simulink model "colab_sim"  (R2023b)
settings: Solver=VariableStepAuto  StartTime=0.0  StopTime=20e-3  RelTol=1e-3
values from neighbouring files (symbols this model uses):
  C = single(10e-6)    [colab_datagen.m]
  dt = 1/f_m    (= 1.25e-06)    [colab_datagen.m]
  ESR = 2    [colab_datagen.m]
  L = single(460e-6)    [colab_datagen.m]
  R = randi([18 50])    [colab_datagen.m]
  R_L = 0.75    [colab_datagen.m]
  Vin = 200    [colab_datagen.m]
libraries: spsSeriesRLCBranchLib x3, spsCurrentMeasurementLib x1, spsDCVoltageSourceLib x1, spsDiodeLib x1, spsMosfetLib x1, dspstat3 x1, dspsrcs4 x1, spsVoltageMeasurementLib x1, spspowerguiLib x1
settings Model: Creator=User  LastModifiedBy=User

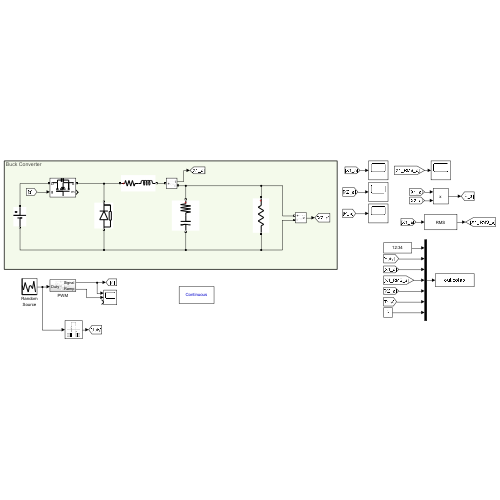
[thumbnail: Simulink's stored preview of the top-level diagram]
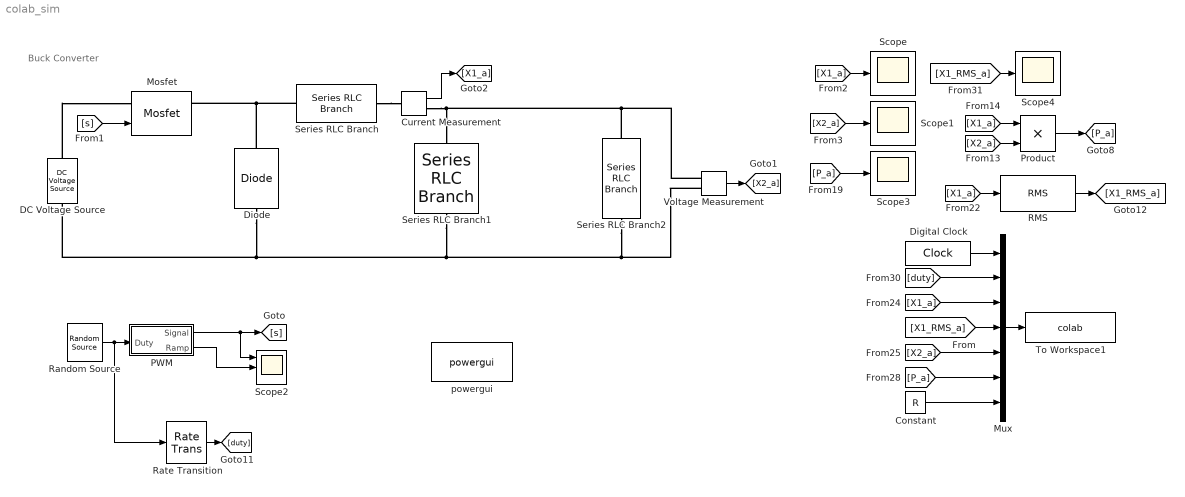
== system colab_sim ==
  note: Buck Converter
  Constant : Constant  Value=R
  Current Measurement : spsCurrentMeasurementLib/Current Measurement  PhasorSimulation=off  OutputType=Complex  PSBequivalent=0
  DC Voltage Source : spsDCVoltageSourceLib/DC Voltage Source  Amplitude=Vin  Measurements=None
  Digital Clock : DigitalClock  SampleTime=dt
  Diode : spsDiodeLib/Diode  Ron=0.1  Lon=0  Vf=VD  IC=0  UseSnubber=0  Rs=500  Cs=250e-9  Measurements=off
  Mosfet : spsMosfetLib/Mosfet  Ron=RDS  Lon=0  Rd=0.1  Vfd=0  IC=0  Rs=1e5  Cs=inf  Measurements=on
  Mux : Mux  Inputs=7
  PWM : Subsystem
  Product : Product
  RMS : dspstat3/RMS  run=off  directionMode=Each column  dimension=1  InputProcessing=Columns as channels (frame based)  reset_popup=None
  Random Source : dspsrcs4/Random Source  SrcType=Uniform  NormMethod=Ziggurat  CltLength=12  MinVal=20  MaxVal=95  MeanVal=0  VarVal=1  RepMode=Not repeatable  rawSeed=1  IsInherit=off  SampMode=Discrete  SampTime=0.005  SampFrame=1  DataType=Double  OutComplex=Real  OutputFrames=off
  Rate Transition : RateTransition  OutPortSampleTime=dt
  Scope{,1,3..4} (4 alike) : Scope
  Scope2 : Scope  NumInputPorts=3
  Series RLC Branch : spsSeriesRLCBranchLib/Series RLC Branch  LConnTagsString=__new0  RConnTagsString=__new0  BranchType=RL  Resistance=R_L  Inductance=L  SetiL0=off  InitialCurrent=0  Capacitance=1e-6  Setx0=off  InitialVoltage=0  Measurements=None
  Series RLC Branch1 : spsSeriesRLCBranchLib/Series RLC Branch  LConnTagsString=__new0  RConnTagsString=__new0  BranchType=RC  Resistance=ESR  Inductance=1e-3  SetiL0=off  InitialCurrent=0  Capacitance=C  Setx0=off  InitialVoltage=0  Measurements=None
  Series RLC Branch2 : spsSeriesRLCBranchLib/Series RLC Branch  LConnTagsString=__new0  RConnTagsString=__new0  BranchType=R  Resistance=R  Inductance=1e-3  SetiL0=off  InitialCurrent=0  Capacitance=1e-6  Setx0=off  InitialVoltage=0  Measurements=None
  To Workspace1 : ToWorkspace  VariableName=colab  SampleTime=-1
  Voltage Measurement : spsVoltageMeasurementLib/Voltage Measurement  PhasorSimulation=off  OutputType=Complex  PSBequivalent=0
  powergui : spspowerguiLib/powergui  Priority=1  SimulationMode=Continuous  SampleTime=1e-6  frequency=60  Iterations=50  frequencyindice=0  Pbase=100e6  ErrMax=1e-4  UnitsV=kV  UnitsW=MW  buscounter=0  FunctionMessages=off  echomessages=off  EnableUseOfTLC=off  CurrentSourceSwitches=off  DisableSnubberDevices=off  DisableRonSwitches=off  DisableVfSwitches=off  DisplayEquations=off  AutomaticDiscreteSolvers=off  SolverType=Tustin/Backward Euler (TBE)  Interpol=off  ExternalGateDelay=off  methode=off  Ts=100  x0status=blocks  SPID=on  SwTol=0  HookPort=off  NonlinearTolerance=1e-4  nMaxIteration=100  ContinueOnMaxIteration=off  RestoreLinks=warning  ResistiveCurrentMeasurement=off  Frange=[0:2:500]  Ylog=off  Xlog=on  ShowGrid=off  save=off  variable=ZData  structure=0  ZoomFFT=off  StartTime=0.0  cycles=1  DisplayStyle=1  fundamental=60  FreqAxis=off  MaxFrequency=1000  frequencyindicesteady=1  RmsSteady=1  display=off
  wires:
  [X2_a] -> Scope1/1
  [s] -> Mosfet/1
  [X1_a] -> Scope/1
  Voltage Measurement/1 -> [X2_a]
  Current Measurement/1 -> [X1_a]
  PWM/1(Signal) -> Scope2/1, [s]
  PWM/2(Ramp) -> Scope2/2
  Random Source/1 -> Rate Transition/1, PWM/1(Duty)
  [X1_a] -> Product/1
  [X2_a] -> Product/2
  Product/1 -> [P_a]
  [P_a] -> Scope3/1
  [X1_a] -> RMS/1
  Rate Transition/1 -> [duty]
  Digital Clock/1 -> Mux/1
  [duty] -> Mux/2
  Mux/1 -> To Workspace1/1
  RMS/1 -> [X1_RMS_a]
  [X1_RMS_a] -> Scope4/1
  [X2_a] -> Mux/5
  [P_a] -> Mux/6
  [X1_a] -> Mux/3
  [X1_RMS_a] -> Mux/4
  Constant/1 -> Mux/7
  connections:
  Diode/RConn1 -- Mosfet/RConn1 -- Series RLC Branch/LConn1
  DC Voltage Source/LConn1 -- Diode/LConn1 -- Voltage Measurement/LConn2 -- Series RLC Branch2/RConn1 -- Series RLC Branch1/RConn1
  Current Measurement/RConn1 -- Series RLC Branch1/LConn1 -- Series RLC Branch2/LConn1 -- Voltage Measurement/LConn1
  Series RLC Branch/RConn1 -- Current Measurement/LConn1
  DC Voltage Source/RConn1 -- Mosfet/LConn1

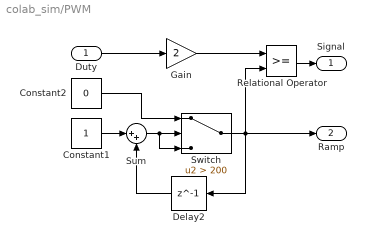
== system colab_sim/PWM ==
  Duty : Inport
  Constant1 : Constant  SampleTime=100e-9
  Constant2 : Constant  Value=0  SampleTime=100e-9
  Delay2 : Delay  DelayLength=1  SampleTime=200e-9
  Gain : Gain  Gain=2
  Relational Operator : RelationalOperator  OutDataTypeStr=boolean  RndMeth=Simplest  InputSameDT=off
  Sum : Sum  Inputs=|++
  Switch : Switch  Criteria=u2 > Threshold  Threshold=200  SaturateOnIntegerOverflow=off  InputSameDT=off
  Signal : Outport
  Ramp : Outport  Port=2
  wires:
  Switch/1 -> Relational Operator/2, Ramp/1, Delay2/1
  Constant2/1 -> Switch/1
  Constant1/1 -> Sum/1
  Sum/1 -> Switch/3, Switch/2
  Delay2/1 -> Sum/2
  Gain/1 -> Relational Operator/1
  Duty/1 -> Gain/1
  Relational Operator/1 -> Signal/1
